simulink model "zadanie3"  (R2016b)
settings: Solver=VariableStepAuto  StartTime=0.0  StopTime=10  RelTol=1e-3
undefined symbols (not defined in the file or in its folder): K1, K2, K3, Tp
settings Model: Creator=michal089  LastModifiedBy=postep

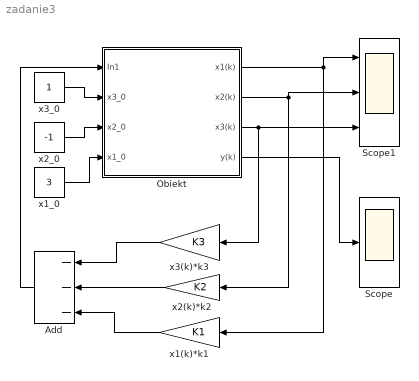
== system zadanie3 ==
  Add : Sum  Inputs=---
  "Obiekt " : Subsystem
  Scope : Scope
  Scope1 : Scope  NumInputPorts=3
  x1(k)*k1 : Gain  Gain=K1
  x1_0 : Constant  Value=3  SampleTime=Tp
  x2(k)*k2 : Gain  Gain=K2
  x2_0 : Constant  Value=-1
  x3(k)*k3 : Gain  Gain=K3
  x3_0 : Constant
  wires:
  x2_0/1 -> "Obiekt "/3(x2_0)
  x3_0/1 -> "Obiekt "/2("x3_0 ")
  x2(k)*k2/1 -> Add/2
  x3(k)*k3/1 -> Add/1
  x1(k)*k1/1 -> Add/3
  "Obiekt "/3(x3(k)) -> x3(k)*k3/1, Scope1/3
  "Obiekt "/2("x2(k) ") -> x2(k)*k2/1, Scope1/2
  "Obiekt "/1("x1(k) ") -> x1(k)*k1/1, Scope1/1
  Add/1 -> "Obiekt "/1(In1)
  x1_0/1 -> "Obiekt "/4(x1_0)
  "Obiekt "/4(y(k)) -> Scope/1

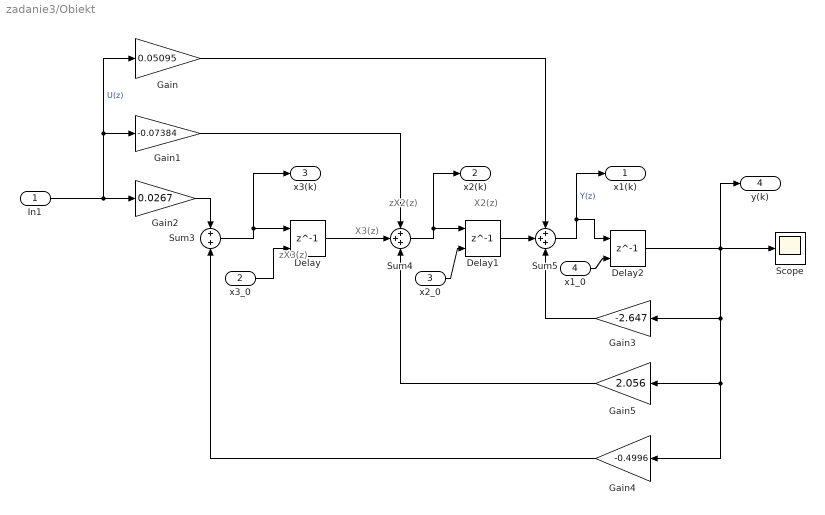
== system zadanie3/Obiekt  ==
  note: X3(z)
  note: zX3(z)
  note: X2(z)
  note: zX2(z)
  In1 : Inport
  "x3_0 " : Inport  Port=2
  x2_0 : Inport  Port=3
  x1_0 : Inport  Port=4
  Delay : Delay  DelayLength=1  InitialConditionSource=Input port  InitialCondition=1  SampleTime=Tp
      settings: InputPortMap=u0,p4
  Delay1 : Delay  DelayLength=1  InitialConditionSource=Input port  InitialCondition=-1  SampleTime=Tp
      settings: InputPortMap=u0,p4
  Delay2 : Delay  DelayLength=1  InitialConditionSource=Input port  InitialCondition=2  SampleTime=Tp
      settings: InputPortMap=u0,p4
  Gain : Gain  Gain=0.05095
  Gain1 : Gain  Gain=-0.07384
  Gain2 : Gain  Gain=0.0267
  Gain3 : Gain  Gain=-2.647
  Gain4 : Gain  Gain=-0.4996
  Gain5 : Gain  Gain=2.056
  Scope : Scope
  Sum3 : Sum
  Sum4 : Sum  Inputs=+++
  Sum5 : Sum  Inputs=+++
  "x1(k) " : Outport
  "x2(k) " : Outport  Port=2
  x3(k) : Outport  Port=3
  y(k) : Outport  Port=4
  wires:
  In1/1 -> Gain/1, Gain1/1, Gain2/1  "U(z)"
  Sum3/1 -> Delay/1, x3(k)/1
  Gain3/1 -> Sum5/3
  Sum5/1 -> Delay2/1, "x1(k) "/1  "Y(z)"
  Gain2/1 -> Sum3/1
  Sum4/1 -> Delay1/1, "x2(k) "/1
  Gain5/1 -> Sum4/3
  Gain4/1 -> Sum3/2
  Gain/1 -> Sum5/1
  Gain1/1 -> Sum4/1
  Delay/1 -> Sum4/2
  "x3_0 "/1 -> Delay/2
  Delay1/1 -> Sum5/2
  x2_0/1 -> Delay1/2
  x1_0/1 -> Delay2/2
  Delay2/1 -> y(k)/1, Scope/1, Gain3/1, Gain5/1, Gain4/1
